simulink model "validacao_dados_degrau"  (R2024a)
settings: Solver=ode45  StartTime=0.0  StopTime=0.7  RelTol=1e-3
values from neighbouring files (symbols this model uses):
  K_degrau = (y_inf)/A    [labeca_02_K_degrau.m]
  tau_area = labeca_02_tau_area()    [labeca_02_simulink_export.m]    (also in labeca_02_tau_area.m = A0/y_inf; labeca_02_validacao_2.m = A0 / y_inf; labeca_02_validacao_26_09.m = A0 / vt_inf)
  tau_nep = labeca_02_tau_neperiano()    [labeca_02_simulink_export.m]    (also in labeca_02_tau_neperiano.m = 1/a; labeca_02_validacao_2.m = 1/a; labeca_02_validacao_26_09.m = 1/a)
settings Model: Creator=Guilherme  LastModifiedBy=Guilherme

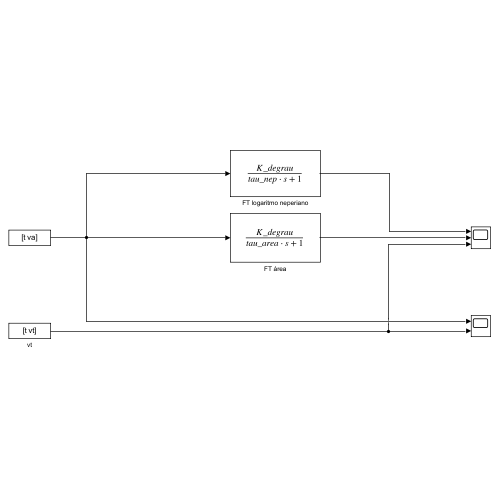
[thumbnail: Simulink's stored preview of the top-level diagram]
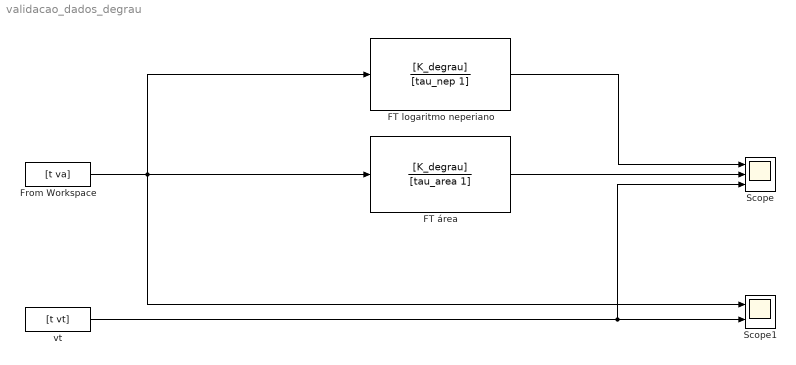
== system validacao_dados_degrau ==
  FT logaritmo neperiano : TransferFcn  Numerator=[K_degrau]  Denominator=[tau_nep 1]
  FT área : TransferFcn  Numerator=[K_degrau]  Denominator=[tau_area 1]
  From Workspace : FromWorkspace  VariableName=[t va]
  Scope : Scope  NumInputPorts=3
  Scope1 : Scope  NumInputPorts=2
  vt : FromWorkspace  VariableName=[t vt]
  wires:
  From Workspace/1 -> Scope1/1, FT área/1, FT logaritmo neperiano/1
  vt/1 -> Scope/3, Scope1/2
  FT área/1 -> Scope/2
  FT logaritmo neperiano/1 -> Scope/1
